simulink model "bike_model_v1_20190531_oldmodel_positionfeedback"  (R2016b)
settings: Solver=ode23s  StartTime=0.0  StopTime=sim_time  FixedStep=Ts_IMU  MaxStep=Ts  RelTol=1e-3
values from neighbouring files (symbols this model uses):
  A = [0      0            1 ... (first row only)    [bike_init_v1_20190528_oldmodel_positionfeedback_and_indicator.m]    (also in bike_init_v1_20190531_oldmodel_positionfeedback_and_indicator.m)
  A_kalman = [1 0 Ts 0; 0 1 0 Ts; 0 0 1 0; 0 0 0 1]    [bike_init_v1_20190528_oldmodel_positionfeedback_and_indicator.m]    (also in bike_init_v1_20190531_oldmodel_positionfeedback_and_indicator.m)
  a_real = b_real-0.77    (= 0.325)    [bike_init_v1_20190528_oldmodel_positionfeedback_and_indicator.m]    (also in bike_init_v1_20190531_oldmodel_positionfeedback_and_indicator.m)
  B = [0; 1; (a_real*v*sin(lambda_real))/(h_real*b_real)]    [bike_init_v1_20190528_oldmodel_positionfeedback_and_indicator.m]    (also in bike_init_v1_20190531_oldmodel_positionfeedback_and_indicator.m)
  B_kalman = [0 0 0 0; 0 0 0 0; 0 0 0 0; 0 0 0 0]    [bike_init_v1_20190528_oldmodel_positionfeedback_and_indicator.m]    (also in bike_init_v1_20190531_oldmodel_positionfeedback_and_indicator.m)
  b_model = 1.095    [bike_init_v1_20190528_oldmodel_positionfeedback_and_indicator.m]    (also in bike_init_v1_20190531_oldmodel_positionfeedback_and_indicator.m)
  b_real = 1.095    [bike_init_v1_20190528_oldmodel_positionfeedback_and_indicator.m]    (also in bike_init_v1_20190531_oldmodel_positionfeedback_and_indicator.m)
  C = eye(3)    [bike_init_v1_20190528_oldmodel_positionfeedback_and_indicator.m]    (also in bike_init_v1_20190531_oldmodel_positionfeedback_and_indicator.m)
  C_kalman = [1 0 0 0; 0 1 0 0; 0 0 1 0; 0 0 0 1]    [bike_init_v1_20190528_oldmodel_positionfeedback_and_indicator.m]    (also in bike_init_v1_20190531_oldmodel_positionfeedback_and_indicator.m)
  complementary = 0.985    [bike_init_v1_20190528_oldmodel_positionfeedback_and_indicator.m]    (also in bike_init_v1_20190531_oldmodel_positionfeedback_and_indicator.m)
  cumulative_dist_along_path = [0;cumsum(dist_from_vertex_to_vertex,1)]    [bike_init_v1_20190528_oldmodel_positionfeedback_and_indicator.m]    (also in bike_init_v1_20190531_oldmodel_positionfeedback_and_indicator.m)
  D = zeros(3,1)    [bike_init_v1_20190528_oldmodel_positionfeedback_and_indicator.m]    (also in bike_init_v1_20190531_oldmodel_positionfeedback_and_indicator.m)
  D_kalman = [0 0 0 0; 0 0 0 0; 0 0 0 0; 0 0 0 0]    [bike_init_v1_20190528_oldmodel_positionfeedback_and_indicator.m]    (also in bike_init_v1_20190531_oldmodel_positionfeedback_and_indicator.m)
  damp = 0.4    [bike_init_v1_20190528_oldmodel_positionfeedback_and_indicator.m]    (also in bike_init_v1_20190531_oldmodel_positionfeedback_and_indicator.m)
  Dead_Band = [0.055,-0.055,0.005]    [bike_init_v1_20190528_oldmodel_positionfeedback_and_indicator.m]    (also in bike_init_v1_20190531_oldmodel_positionfeedback_and_indicator.m)
  delay = 0.045    [bike_init_v1_20190528_oldmodel_positionfeedback_and_indicator.m]    (also in bike_init_v1_20190531_oldmodel_positionfeedback_and_indicator.m)
  delta_control = 1    [bike_init_v1_20190528_oldmodel_positionfeedback_and_indicator.m]    (also in bike_init_v1_20190531_oldmodel_positionfeedback_and_indicator.m)
  direct_control = 1    [bike_init_v1_20190528_oldmodel_positionfeedback_and_indicator.m]    (also in bike_init_v1_20190531_oldmodel_positionfeedback_and_indicator.m)
  filter_model = 1    [bike_init_v1_20190528_oldmodel_positionfeedback_and_indicator.m]    (also in bike_init_v1_20190531_oldmodel_positionfeedback_and_indicator.m)
  forward_motor_dynamics = 0    [bike_init_v1_20190528_oldmodel_positionfeedback_and_indicator.m]    (also in bike_init_v1_20190531_oldmodel_positionfeedback_and_indicator.m)
  fr_oscil = 1    [bike_init_v1_20190528_oldmodel_positionfeedback_and_indicator.m]    (also in bike_init_v1_20190531_oldmodel_positionfeedback_and_indicator.m)
  g = 9.81    [bike_init_v1_20190528_oldmodel_positionfeedback_and_indicator.m]    (also in bike_init_v1_20190531_oldmodel_positionfeedback_and_indicator.m)
  gain = 0.3    [bike_init_v1_20190528_oldmodel_positionfeedback_and_indicator.m]    (also in bike_init_v1_20190531_oldmodel_positionfeedback_and_indicator.m)
  h_real = 0.586    [bike_init_v1_20190528_oldmodel_positionfeedback_and_indicator.m]    (also in bike_init_v1_20190531_oldmodel_positionfeedback_and_indicator.m)
  IMU_height_model = 0.45    [bike_init_v1_20190528_oldmodel_positionfeedback_and_indicator.m]    (also in bike_init_v1_20190531_oldmodel_positionfeedback_and_indicator.m)
  IMU_height_real = 0.45    [bike_init_v1_20190528_oldmodel_positionfeedback_and_indicator.m]    (also in bike_init_v1_20190531_oldmodel_positionfeedback_and_indicator.m)
  initial_states = [deg2rad(0) deg2rad(0) deg2rad(0)]    [bike_init_v1_20190528_oldmodel_positionfeedback_and_indicator.m]    (also in bike_init_v1_20190531_oldmodel_positionfeedback_and_indicator.m = [deg2rad(2) deg2rad(0) deg2rad(0)])
  initial_x = path_x(1)+x_ini_diff    [bike_init_v1_20190528_oldmodel_positionfeedback_and_indicator.m]    (also in bike_init_v1_20190531_oldmodel_positionfeedback_and_indicator.m = 0)
  initial_y = radius+y_ini_diff    (= 20)    [bike_init_v1_20190528_oldmodel_positionfeedback_and_indicator.m]    (also in bike_init_v1_20190531_oldmodel_positionfeedback_and_indicator.m = 0)
  input_velocity = 7    [bike_init_v1_20190528_oldmodel_positionfeedback_and_indicator.m]    (also in bike_init_v1_20190531_oldmodel_positionfeedback_and_indicator.m = 3)
  K_full_dis = zeros(length(velocity_lqr),3)    [bike_init_v1_20190528_oldmodel_positionfeedback_and_indicator.m]    (also in bike_init_v1_20190531_oldmodel_positionfeedback_and_indicator.m)
  lambda_model = deg2rad(70)    [bike_init_v1_20190528_oldmodel_positionfeedback_and_indicator.m]    (also in bike_init_v1_20190531_oldmodel_positionfeedback_and_indicator.m)
  lambda_real = deg2rad(70)    [bike_init_v1_20190528_oldmodel_positionfeedback_and_indicator.m]    (also in bike_init_v1_20190531_oldmodel_positionfeedback_and_indicator.m)
  lat_control = 1    [bike_init_v1_20190528_oldmodel_positionfeedback_and_indicator.m]    (also in bike_init_v1_20190531_oldmodel_positionfeedback_and_indicator.m)
  look_ahead = 0    [bike_init_v1_20190528_oldmodel_positionfeedback_and_indicator.m]    (also in bike_init_v1_20190531_oldmodel_positionfeedback_and_indicator.m)
  max_handlebar = 40*(pi/180)    (= 0.698131700798)    [bike_init_v1_20190528_oldmodel_positionfeedback_and_indicator.m]    (also in bike_init_v1_20190531_oldmodel_positionfeedback_and_indicator.m)
  max_roll = pi/2    (= 1.57079632679)    [bike_init_v1_20190528_oldmodel_positionfeedback_and_indicator.m]    (also in bike_init_v1_20190531_oldmodel_positionfeedback_and_indicator.m)
  max_steering_motor_acc = inf    [bike_init_v1_20190528_oldmodel_positionfeedback_and_indicator.m]    (also in bike_init_v1_20190531_oldmodel_positionfeedback_and_indicator.m)
  max_steering_motor_speed = 7.5    [bike_init_v1_20190528_oldmodel_positionfeedback_and_indicator.m]    (also in bike_init_v1_20190531_oldmodel_positionfeedback_and_indicator.m)
  min_handlebar = -max_handlebar    (= -0.698131700798)    [bike_init_v1_20190528_oldmodel_positionfeedback_and_indicator.m]    (also in bike_init_v1_20190531_oldmodel_positionfeedback_and_indicator.m)
  min_roll = - max_roll    (= -1.57079632679)    [bike_init_v1_20190528_oldmodel_positionfeedback_and_indicator.m]    (also in bike_init_v1_20190531_oldmodel_positionfeedback_and_indicator.m)
  min_steering_motor_acc = -inf    [bike_init_v1_20190528_oldmodel_positionfeedback_and_indicator.m]    (also in bike_init_v1_20190531_oldmodel_positionfeedback_and_indicator.m)
  min_steering_motor_speed = -7.5    [bike_init_v1_20190528_oldmodel_positionfeedback_and_indicator.m]    (also in bike_init_v1_20190531_oldmodel_positionfeedback_and_indicator.m)
  noise = 1    [bike_init_v1_20190528_oldmodel_positionfeedback_and_indicator.m]    (also in bike_init_v1_20190531_oldmodel_positionfeedback_and_indicator.m)
  noise_encoder = 1e-7    (= 1e-07)    [bike_init_v1_20190528_oldmodel_positionfeedback_and_indicator.m]    (also in bike_init_v1_20190531_oldmodel_positionfeedback_and_indicator.m)
  noise_hall = 0.01    [bike_init_v1_20190528_oldmodel_positionfeedback_and_indicator.m]    (also in bike_init_v1_20190531_oldmodel_positionfeedback_and_indicator.m = 0.0031)
  noise_pos_meas = 0.51    [bike_init_v1_20190528_oldmodel_positionfeedback_and_indicator.m]    (also in bike_init_v1_20190531_oldmodel_positionfeedback_and_indicator.m)
  oscillations_roll = 0    [bike_init_v1_20190528_oldmodel_positionfeedback_and_indicator.m]    (also in bike_init_v1_20190531_oldmodel_positionfeedback_and_indicator.m)
  oscillations_steer = 0    [bike_init_v1_20190528_oldmodel_positionfeedback_and_indicator.m]    (also in bike_init_v1_20190531_oldmodel_positionfeedback_and_indicator.m)
  parameters_model = [g h_model b_model a_model lambda_model c_model]    [bike_init_v1_20190528_oldmodel_positionfeedback_and_indicator.m]    (also in bike_init_v1_20190531_oldmodel_positionfeedback_and_indicator.m)
  parameters_real = [g h_real b_real a_real lambda_real c_real]    [bike_init_v1_20190528_oldmodel_positionfeedback_and_indicator.m]    (also in bike_init_v1_20190531_oldmodel_positionfeedback_and_indicator.m)
  path_tracking = 0    [bike_init_v1_20190528_oldmodel_positionfeedback_and_indicator.m]    (also in bike_init_v1_20190531_oldmodel_positionfeedback_and_indicator.m)
  path_x = [path_x1 path_x2 path_x3]    [bike_init_v1_20190528_oldmodel_positionfeedback_and_indicator.m]    (also in bike_init_v1_20190531_oldmodel_positionfeedback_and_indicator.m)
  path_y = [path_y1 path_y2 path_y3]    [bike_init_v1_20190528_oldmodel_positionfeedback_and_indicator.m]    (also in bike_init_v1_20190531_oldmodel_positionfeedback_and_indicator.m)
  plant_model = 1    [bike_init_v1_20190528_oldmodel_positionfeedback_and_indicator.m]    (also in bike_init_v1_20190531_oldmodel_positionfeedback_and_indicator.m)
  R_kalman = [noise_pos_meas 0 0 0; 0 noise_pos_meas 0 0; 0 0 noise_hall 0; 0 0 0 noise_hall]    [bike_init_v1_20190528_oldmodel_positionfeedback_and_indicator.m]    (also in bike_init_v1_20190531_oldmodel_positionfeedback_and_indicator.m)
  roll_rate_coef = 0.9    [bike_init_v1_20190528_oldmodel_positionfeedback_and_indicator.m]    (also in bike_init_v1_20190531_oldmodel_positionfeedback_and_indicator.m)
  steering_motor_limitations = 1    [bike_init_v1_20190528_oldmodel_positionfeedback_and_indicator.m]    (also in bike_init_v1_20190531_oldmodel_positionfeedback_and_indicator.m)
  sys_con = ss(A,B,C,D)    [bike_init_v1_20190528_oldmodel_positionfeedback_and_indicator.m]    (also in bike_init_v1_20190531_oldmodel_positionfeedback_and_indicator.m)
  sys_dis = c2d(sys_con,Ts)    [bike_init_v1_20190528_oldmodel_positionfeedback_and_indicator.m]    (also in bike_init_v1_20190531_oldmodel_positionfeedback_and_indicator.m)
  Ts = 0.04    [bike_init_v1_20190528_oldmodel_positionfeedback_and_indicator.m]    (also in bike_init_v1_20190531_oldmodel_positionfeedback_and_indicator.m)
  Ts_IMU = 0.04    [bike_init_v1_20190528_oldmodel_positionfeedback_and_indicator.m]    (also in bike_init_v1_20190531_oldmodel_positionfeedback_and_indicator.m)
  velocity_lqr = [velocity_lqr-0.1 velocity_lqr velocity_lqr+0.1]    [bike_init_v1_20190528_oldmodel_positionfeedback_and_indicator.m]    (also in bike_init_v1_20190531_oldmodel_positionfeedback_and_indicator.m)
  velocity_wave_amp = 0.5    [bike_init_v1_20190528_oldmodel_positionfeedback_and_indicator.m]    (also in bike_init_v1_20190531_oldmodel_positionfeedback_and_indicator.m)
  velocity_wave_freq = 0.3*2*pi    (= 1.88495559215)    [bike_init_v1_20190528_oldmodel_positionfeedback_and_indicator.m]    (also in bike_init_v1_20190531_oldmodel_positionfeedback_and_indicator.m)
undefined symbols (not defined in the file or in its folder): Continuous, curvature, Time
libraries: simulink x13, mpclib x2, dspsigops x2, simulink_extras x1, ctrlSharedLib x1
(part 1 of 2)
settings Model: Creator=Boaz Ash  LastModifiedBy=maximefeingesicht
settings DebuggingCC: UnconnectedInputMsg=none  UnconnectedOutputMsg=none  UnconnectedLineMsg=none

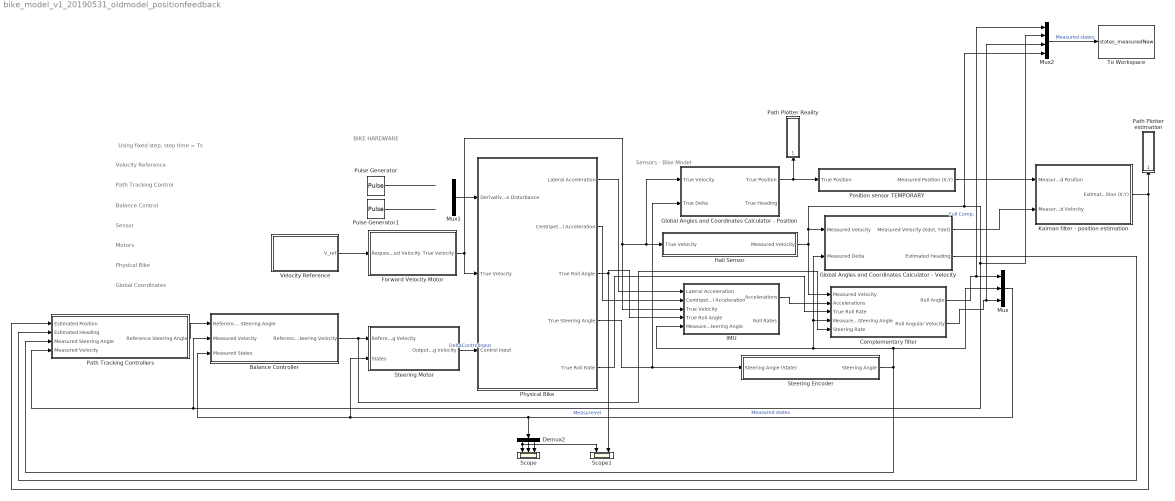
== system bike_model_v1_20190531_oldmodel_positionfeedback ==
  note: Using fixed step, step time = Ts
  note: BIKE HARDWARE
  note: Velocity Reference
  note: Sensor
  note: Sensors - Bike Model
  note: Balance Control
  note: Motors
  note: Physical Bike
  note: Path Tracking Control
  note: Global Coordinates
  Balance Controller : Subsystem  TreatAsAtomicUnit=on  SystemSampleTime=Ts
  Complementary filter : Subsystem  SystemSampleTime=Ts_IMU
  Demux2 : Demux  Outputs=3
  Forward Velocity Motor : Subsystem
  Global Angles and Coordinates Calculator - Position : Subsystem  SystemSampleTime=Ts
  Global Angles and Coordinates Calculator - Velocity : Subsystem  SystemSampleTime=Ts
  Hall Sensor : Subsystem  TreatAsAtomicUnit=on  SystemSampleTime=Ts
  IMU : Subsystem  TreatAsAtomicUnit=on
  "Kalman filter - position estimation " : Subsystem  SystemSampleTime=Ts
  Mux : Mux  Inputs=3
  Mux1 : Mux  Inputs=3
  Mux2 : Mux
  Path Plotter Reality : Subsystem  SystemSampleTime=Ts
  Path Plotter estimation : Subsystem  SystemSampleTime=Ts
  Path Tracking Controllers : Subsystem
  Physical Bike : Subsystem
  Position sensor TEMPORARY : Subsystem  TreatAsAtomicUnit=on  SystemSampleTime=Ts
  Pulse Generator : DiscretePulseGenerator  PulseType=Time based  Amplitude=pi/36  Period=100  PhaseDelay=1
  Pulse Generator1 : DiscretePulseGenerator  PulseType=Time based  Amplitude=-deg2rad(30)  Period=10  PulseWidth=10  PhaseDelay=1
  Scope : Scope  NumInputPorts=3
  Scope1 : Scope  NumInputPorts=2
  Steering Encoder : Subsystem  TreatAsAtomicUnit=on  SystemSampleTime=Ts
  Steering Motor : Subsystem
  To Workspace : ToWorkspace  VariableName=states_measuredNew  SaveFormat=Timeseries  SampleTime=-1
  Velocity Reference : Subsystem
  wires:
  Mux1/1 -> Physical Bike/1(Derivative Disturbance)
  Velocity Reference/1(V_ref) -> Forward Velocity Motor/1(Requested Velocity)
  Demux2/2 -> Scope/2
  Demux2/3 -> Scope/3
  Forward Velocity Motor/1(True Velocity) -> IMU/3(True Velocity), Global Angles and Coordinates Calculator - Position/1(True Velocity), Hall Sensor/1(True Velocity), Physical Bike/2(True Velocity)
  Pulse Generator/1 -> ?
  Physical Bike/4(True Steering Angle) -> Global Angles and Coordinates Calculator - Position/2(True Delta), Steering Encoder/1(Steering Angle (State))
  Pulse Generator1/1 -> ?
  "Kalman filter - position estimation "/1(Estimated Position (X,Y)) -> Path Tracking Controllers/1(Estimated Position), Path Plotter estimation/1(Position)
  Global Angles and Coordinates Calculator - Velocity/2(Estimated Heading) -> Path Tracking Controllers/2(Estimated Heading)
  Path Tracking Controllers/1(Reference Steering Angle) -> Balance Controller/1(Reference Steering Angle)
  Balance Controller/1(Reference Steering Velocity) -> Complementary filter/5(Steering Rate), Steering Motor/1(Reference Steering Velocity)
  Demux2/1 -> Scope1/1, Scope/1
  Physical Bike/1(Lateral Acceleration) -> IMU/1(Lateral Acceleration)
  Physical Bike/2(Centripetal Acceleration) -> IMU/2(Centripetal Acceleration)
  Mux/1 -> Demux2/1, Steering Motor/2(States), Balance Controller/3(Measured States)  "Measured states"
  Physical Bike/5(True Roll Rate) -> Complementary filter/3(True Roll Rate)
  Physical Bike/3(True Roll Angle) -> IMU/4(True Roll Angle), Scope1/2
  Steering Motor/1(Output Steering Velocity) -> Physical Bike/3(Control Input)  "DeltaControlInput"
  Steering Encoder/1(Steering Angle) -> Global Angles and Coordinates Calculator - Velocity/2(Measured Delta), Complementary filter/4(Measured Steering Angle), IMU/5(Measured Steering Angle), Mux/2, Path Tracking Controllers/3(Measured Steering Angle)
  IMU/1(Accelerations) -> Complementary filter/2(Accelerations)
  Position sensor TEMPORARY/1("Measured Position (X,Y) ") -> "Kalman filter - position estimation "/1("Measured Position ")
  Global Angles and Coordinates Calculator - Position/1(True Position) -> Path Plotter Reality/1(Position), Position sensor TEMPORARY/1(True Position)
  Global Angles and Coordinates Calculator - Velocity/1("Measured Velocity (Xdot, Ydot)") -> "Kalman filter - position estimation "/2(Measured Velocity)
  Complementary filter/2(Roll Angular Velocity) -> Mux2/3, Mux/3
  Complementary filter/1(Roll Angle) -> Mux2/1, Mux/1  "Full Comp."
  Hall Sensor/1(Measured Velocity) -> Mux2/4, Path Tracking Controllers/4(Measured Velocity), Balance Controller/2(Measured Velocity), Mux2/2, Global Angles and Coordinates Calculator - Velocity/1(Measured Velocity), Complementary filter/1(Measured Velocity)  "MeasureVel"
  Mux2/1 -> To Workspace/1  "Measured states"

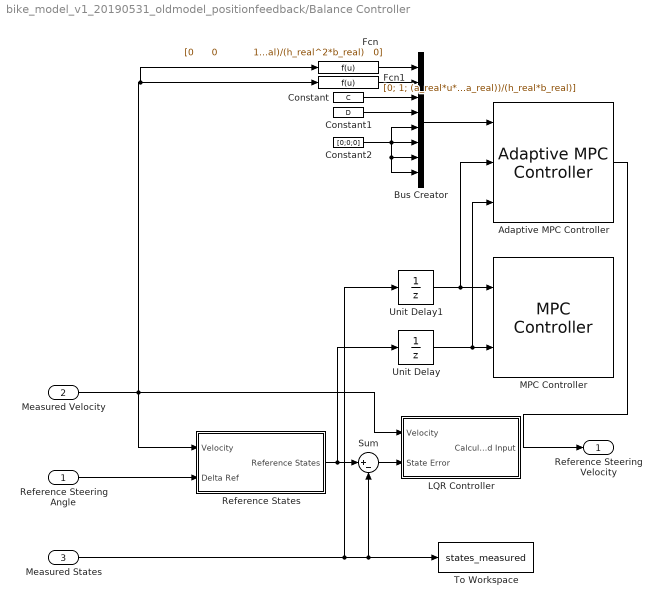
== system bike_model_v1_20190531_oldmodel_positionfeedback/Balance Controller ==
  Reference Steering Angle : Inport
  Measured Velocity : Inport  Port=2
  Measured States : Inport  Port=3
  Adaptive MPC Controller : mpclib/Adaptive MPC Controller  SCDEnableBlockLinearizationSpecification=on  mpcobj=mpcObj  md_inport=off  mv_inport=off  cost_outport=off  return_sequence=off  return_qpstatus=off  return_state=off  state_inport=off  isltv_plant=off  lims_inport=off  ywt_inport=off  uwt_inport=off  duwt_inport=off  rhoeps_inport=off  uref_inport=off  BlockDataType=double  SampleTimeInherited=off  switch_inport=off
  Bus Creator : BusCreator  Inputs='A','B','C','D','X','Y','U','DX'
  Constant : Constant  Value=C  SampleTime=Ts
  Constant1 : Constant  Value=D  SampleTime=Ts
  Constant2 : Constant  Value=[0;0;0]  SampleTime=Ts
  Fcn : Fcn  Expr=|
      | [0      0            1;
      |              0      0            0;
      |              g/h_real    sin(lambda_real)*(h_real*u^2-g*a_real*c_real)/(h_real^2*b_real)   0]
  Fcn1 : Fcn  Expr=[0; 1; (a_real*u*sin(lambda_real))/(h_real*b_real)]
  LQR Controller : Subsystem  TreatAsAtomicUnit=on  SystemSampleTime=Ts
  MPC Controller : mpclib/MPC Controller  SCDEnableBlockLinearizationSpecification=on  mpcobj=mpcObj  is_multiple=0  enable_value=0  return_u0=off  ref_from_ws=off  ref_signal_name=[]  ref_preview=off  md_from_ws=off  md_signal_name=[]  md_preview=off  from_project=off  project_file=MPCtask.mat  md_inport=off  mv_inport=off  cost_outport=off  return_sequence=off  return_qpstatus=off  return_state=off  state_inport=off  lims_inport=off  ywt_inport=off  is_designfromscratch=0  uwt_inport=off  duwt_inport=off  rhoeps_inport=off  uref_inport=off  n_ts=0.04  n_mv=1  n_md=0  n_ud=0  n_mo=3  n_uo=0  BlockDataType=double  SampleTimeInherited=off  switch_inport=off
  Reference States : Subsystem  SystemSampleTime=Ts
  Sum : Sum  Inputs=|+-
  To Workspace : ToWorkspace  VariableName=states_measured  SaveFormat=Timeseries  SampleTime=-1
  Unit Delay : UnitDelay  InitialCondition=[0 0 0]  SampleTime=-1
  Unit Delay1 : UnitDelay  InitialCondition=[0 0 0]  SampleTime=-1
  Reference Steering Velocity : Outport
  wires:
  Reference States/1(Reference States) -> Unit Delay/1, Sum/1
  Sum/1 -> LQR Controller/2(State Error)
  Adaptive MPC Controller/1 -> Reference Steering Velocity/1
  Reference Steering Angle/1 -> Reference States/2(Delta Ref)
  Measured Velocity/1 -> Fcn/1, Fcn1/1, Reference States/1(Velocity), LQR Controller/1(Velocity)
  Unit Delay/1 -> Adaptive MPC Controller/3, MPC Controller/2
  Measured States/1 -> Unit Delay1/1, To Workspace/1, Sum/2
  Unit Delay1/1 -> Adaptive MPC Controller/2, MPC Controller/1
  Bus Creator/1 -> Adaptive MPC Controller/1
  Fcn1/1 -> Bus Creator/2
  Fcn/1 -> Bus Creator/1
  Constant/1 -> Bus Creator/3
  Constant1/1 -> Bus Creator/4
  Constant2/1 -> Bus Creator/7, Bus Creator/8, Bus Creator/6, Bus Creator/5

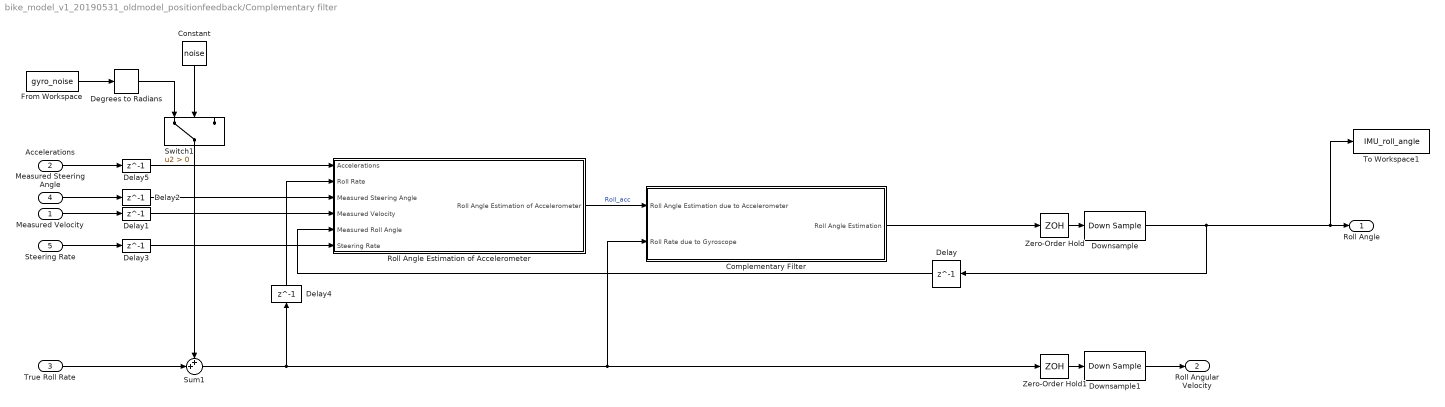
== system bike_model_v1_20190531_oldmodel_positionfeedback/Complementary filter ==
  Measured Velocity : Inport
  Accelerations : Inport  Port=2
  True Roll Rate : Inport  Port=3
  Measured Steering Angle : Inport  Port=4
  Steering Rate : Inport  Port=5
  Complementary Filter : Subsystem  TreatAsAtomicUnit=on  SystemSampleTime=Ts_IMU
  Constant : Constant  Value=noise
  Degrees to Radians : simulink_extras/Transformations/Degrees to Radians
  Delay{,1..2,4..5} (5 alike) : Delay  DelayLength=1
  Delay3 : Delay  DelayLength=1  SampleTime=Ts_IMU
  Downsample : DownSample  N=Ts/Ts_IMU  RateOptions=Allow multirate processing
  Downsample1 : DownSample  N=Ts/Ts_IMU  RateOptions=Allow multirate processing
  From Workspace : FromWorkspace  VariableName=gyro_noise  SampleTime=0
  Roll Angle Estimation of Accelerometer : Subsystem
  Sum1 : Sum  Inputs=++|
  Switch1 : Switch  Criteria=u2 > Threshold
  To Workspace1 : ToWorkspace  VariableName=IMU_roll_angle  SaveFormat=Structure  SampleTime=-1
  Zero-Order Hold : ZeroOrderHold  SampleTime=Ts_IMU
  Zero-Order Hold1 : ZeroOrderHold  SampleTime=Ts_IMU
  Roll Angle : Outport
  Roll Angular Velocity : Outport  Port=2
  wires:
  Constant/1 -> Switch1/2
  True Roll Rate/1 -> Sum1/2
  Roll Angle Estimation of Accelerometer/1(Roll Angle Estimation of Accelerometer) -> Complementary Filter/1(Roll Angle Estimation due to Accelerometer)  "Roll_acc"
  Switch1/1 -> Sum1/1
  Sum1/1 -> Zero-Order Hold1/1, Complementary Filter/2(Roll Rate due to Gyroscope), Delay4/1
  Zero-Order Hold/1 -> Downsample/1
  Zero-Order Hold1/1 -> Downsample1/1
  Accelerations/1 -> Delay5/1
  Measured Steering Angle/1 -> Delay2/1
  Measured Velocity/1 -> Delay1/1
  Delay/1 -> Roll Angle Estimation of Accelerometer/5(Measured Roll Angle)
  Delay1/1 -> Roll Angle Estimation of Accelerometer/4(Measured Velocity)
  Delay2/1 -> Roll Angle Estimation of Accelerometer/3(Measured Steering Angle)
  Steering Rate/1 -> Delay3/1
  Delay3/1 -> Roll Angle Estimation of Accelerometer/6(Steering Rate)
  Delay4/1 -> Roll Angle Estimation of Accelerometer/2(Roll Rate)
  Delay5/1 -> Roll Angle Estimation of Accelerometer/1(Accelerations)
  Complementary Filter/1(Roll Angle Estimation) -> Zero-Order Hold/1
  From Workspace/1 -> Degrees to Radians/1
  Degrees to Radians/1 -> Switch1/1
  Downsample1/1 -> Roll Angular Velocity/1
  Downsample/1 -> To Workspace1/1, Roll Angle/1, Delay/1

== system bike_model_v1_20190531_oldmodel_positionfeedback/Forward Velocity Motor ==
  note: Add limit for acceleration/deceleration
      | Add min speed of 1.69 m/s (3600 rpm motor speed) limitation
      | Add min speed of 8.20 m/s (18000 rpm motor speed) limitation
      | Add deadband and delay
  Requested Velocity : Inport
  Constant : Constant  Value=forward_motor_dynamics
  Rate Limiter : RateLimiter  RisingSlewLimit=inf  FallingSlewLimit=-inf  SampleTimeMode=inherited
  Saturation : Saturate  UpperLimit=inf  LowerLimit=0
  Scope : Scope
  Sine Wave : Sin  Amplitude=velocity_wave_amp  Frequency=velocity_wave_freq  SampleTime=0
  Sum : Sum  Inputs=|++
  Switch : Switch  Criteria=u2 > Threshold
  Transfer Fcn : TransferFcn  Numerator=[-0.2156 0.556]  Denominator=[1 1.675 0.5558]
  True Velocity : Outport
  wires:
  Requested Velocity/1 -> Transfer Fcn/1, Switch/3
  Transfer Fcn/1 -> Rate Limiter/1
  Switch/1 -> Sum/1
  Constant/1 -> Switch/2
  Saturation/1 -> Switch/1
  Rate Limiter/1 -> Saturation/1
  Sum/1 -> Scope/1, True Velocity/1
  Sine Wave/1 -> Sum/2

== system bike_model_v1_20190531_oldmodel_positionfeedback/Global Angles and Coordinates Calculator - Position ==
  True Velocity : Inport
  True Delta : Inport  Port=2
  Gain1 : Gain  Gain=sin(lambda_model)
  Measured Bike Angles to Global Angles : Subsystem
  Measured Global Angles to Global Coordinates : Subsystem
  Sum : Sum  Inputs=++|
  To Workspace : ToWorkspace  VariableName=pos_true  SaveFormat=Timeseries  SampleTime=-1
  True Position : Outport
  True Heading : Outport  Port=2
  wires:
  True Delta/1 -> Gain1/1
  Measured Bike Angles to Global Angles/1(psi) -> Sum/2, Measured Global Angles to Global Coordinates/2(Psi)
  Gain1/1 -> Measured Bike Angles to Global Angles/2(Steering Angle)
  Sum/1 -> True Heading/1
  Measured Bike Angles to Global Angles/2(beta) -> Sum/1, Measured Global Angles to Global Coordinates/3(Beta)
  Measured Global Angles to Global Coordinates/1("Position (X, Y)") -> To Workspace/1, True Position/1
  True Velocity/1 -> Measured Bike Angles to Global Angles/1(Velocity), Measured Global Angles to Global Coordinates/1(Velocity)

== system bike_model_v1_20190531_oldmodel_positionfeedback/Global Angles and Coordinates Calculator - Velocity ==
  Measured Velocity : Inport
  Measured Delta : Inport  Port=2
  Gain1 : Gain  Gain=sin(lambda_model)
  Integrator2 : Integrator
  Measured Bike Angles to Global Angles : Subsystem
  Measured Global Angles to Global Coordinates : Subsystem
  Sum : Sum  Inputs=++|
  To Workspace1 : ToWorkspace  VariableName=pos_vel_int  SaveFormat=Timeseries  SampleTime=-1
  "Measured Velocity (Xdot, Ydot)" : Outport
  Estimated Heading : Outport  Port=2
  wires:
  Measured Delta/1 -> Gain1/1
  Measured Bike Angles to Global Angles/1(psi) -> Sum/2, Measured Global Angles to Global Coordinates/2(Psi)
  Gain1/1 -> Measured Bike Angles to Global Angles/2(Steering Angle)
  Sum/1 -> Estimated Heading/1
  Measured Bike Angles to Global Angles/2(beta) -> Measured Global Angles to Global Coordinates/3(Beta), Sum/1
  Measured Velocity/1 -> Measured Bike Angles to Global Angles/1(Velocity), Measured Global Angles to Global Coordinates/1(Velocity)
  Measured Global Angles to Global Coordinates/1("Velocity (Xdot, Ydot)") -> Integrator2/1, "Measured Velocity (Xdot, Ydot)"/1
  Integrator2/1 -> To Workspace1/1

== system bike_model_v1_20190531_oldmodel_positionfeedback/Hall Sensor ==
  True Velocity : Inport
  Constant : Constant  Value=noise
  Noise on hall sensor : RandomNumber  Variance=noise_hall  SampleTime=Ts
  Saturate Signal : Switch  Criteria=u2 > Threshold
  Sum : Sum  Inputs=++|
  Switch : Switch  Criteria=u2 > Threshold
  To Workspace3 : ToWorkspace  VariableName=vel_meas  SaveFormat=Timeseries  SampleTime=-1
  Velocity Lower Bound : simulink/Model Verification/Check Static  Lower Bound  Description=0.6 <= u  min=0.6  min_included=on  enabled=on  stopWhenAssertionFail=off  export=on  icon=graphic
  Zero : Constant  Value=0
  Zero-Order Hold : ZeroOrderHold  SampleTime=Ts
  Measured Velocity : Outport
  wires:
  Constant/1 -> Switch/2
  Switch/1 -> Saturate Signal/1, Velocity Lower Bound/1
  Noise on hall sensor/1 -> Sum/1
  Sum/1 -> Switch/1
  Zero/1 -> Saturate Signal/3
  Velocity Lower Bound/1 -> Saturate Signal/2
  Saturate Signal/1 -> Zero-Order Hold/1
  Zero-Order Hold/1 -> Measured Velocity/1, To Workspace3/1
  True Velocity/1 -> Switch/3, Sum/2

== system bike_model_v1_20190531_oldmodel_positionfeedback/IMU ==
  Lateral Acceleration : Inport
  Centripetal Acceleration : Inport  Port=2
  True Velocity : Inport  Port=3
  True Roll Angle : Inport  Port=4
  Measured Steering Angle : Inport  Port=5
  IMU : Subsystem
  Accelerations : Outport
  Roll Rates : Outport  Port=2
  wires:
  True Velocity/1 -> IMU/3(True Velocity)
  True Roll Angle/1 -> IMU/4(True Roll Angle)
  Measured Steering Angle/1 -> IMU/5(Measured Steering Angle)
  Lateral Acceleration/1 -> IMU/1(Lateral Acceleration)
  Centripetal Acceleration/1 -> IMU/2(Centripetal Acceleration)
  IMU/1(Accelerations) -> Accelerations/1
  IMU/2(Roll Rates) -> Roll Rates/1

== system bike_model_v1_20190531_oldmodel_positionfeedback/Kalman filter - position estimation  ==
  note: y_k
  note: Measurements
  "Measured Position " : Inport
  Measured Velocity : Inport  Port=2
  Demux : Demux  Outputs=2
  "Kalman Filter " : ctrlSharedLib/Kalman Filter  TimeDomain=Continuous-Time  UseCurrentEstimator=on  ModelSource=Individual A, B, C, D matrices  ModelSourceVariable=ss(0.95,1,1,0,1)  A=A_kalman  B=B_kalman  C=C_kalman  D=D_kalman  NumberOfStates=1  NumberOfInputs=1  NumberOfOutputs=1  InitialEstimateSource=Dialog  X0=0  P0=10  UseK=off  UseGH=off  NumberOfProcessNoiseInputs=1  G=1  TimeInvariantG=on  H=0  TimeInvariantH=on  Q=Q_kalman  TimeInvariantQ=on  R=R_kalman  TimeInvariantR=on  N=0  TimeInvariantN=on  AddInputPort=on  AddEnablePort=off  ExternalReset=none  OutputEstimatedY=off  OutputP=off  Ts=Ts
  Mux : Mux  Inputs=2
  Estimated Position (X,Y) : Outport
  wires:
  Measured Velocity/1 -> Mux/2
  Mux/1 -> "Kalman Filter "/2
  "Measured Position "/1 -> Mux/1
  "Kalman Filter "/1 -> Demux/1
  Demux/1 -> Estimated Position (X,Y)/1

== system bike_model_v1_20190531_oldmodel_positionfeedback/Path Plotter Reality ==
  Position : Inport
  Demux : Demux  Outputs=2
  To Workspace : ToWorkspace  VariableName=X_BIKE  SaveFormat=Timeseries  SampleTime=Ts
  To Workspace1 : ToWorkspace  VariableName=Y_BIKE  SaveFormat=Timeseries  SampleTime=Ts
  XY Graph : simulink/Sinks/XY Graph  Commented=on  xmin=min(path_x)-5  xmax=max(path_x)+5  ymin=min(path_y)-5  ymax=max(path_y)+5  st=-1
  wires:
  Demux/1 -> XY Graph/1, To Workspace/1  "X"
  Demux/2 -> XY Graph/2, To Workspace1/1  "Y"
  Position/1 -> Demux/1

== system bike_model_v1_20190531_oldmodel_positionfeedback/Path Plotter estimation ==
  Position : Inport
  Demux : Demux  Outputs=2
  To Workspace : ToWorkspace  VariableName=X_BIKE_estim  SaveFormat=Timeseries  SampleTime=Ts
  To Workspace1 : ToWorkspace  VariableName=Y_BIKE_estim  SaveFormat=Timeseries  SampleTime=Ts
  XY Graph : simulink/Sinks/XY Graph  Commented=on  xmin=min(path_x)-5  xmax=max(path_x)+5  ymin=min(path_y)-5  ymax=max(path_y)+5  st=-1
  wires:
  Demux/1 -> XY Graph/1, To Workspace/1  "X"
  Demux/2 -> XY Graph/2, To Workspace1/1  "Y"
  Position/1 -> Demux/1

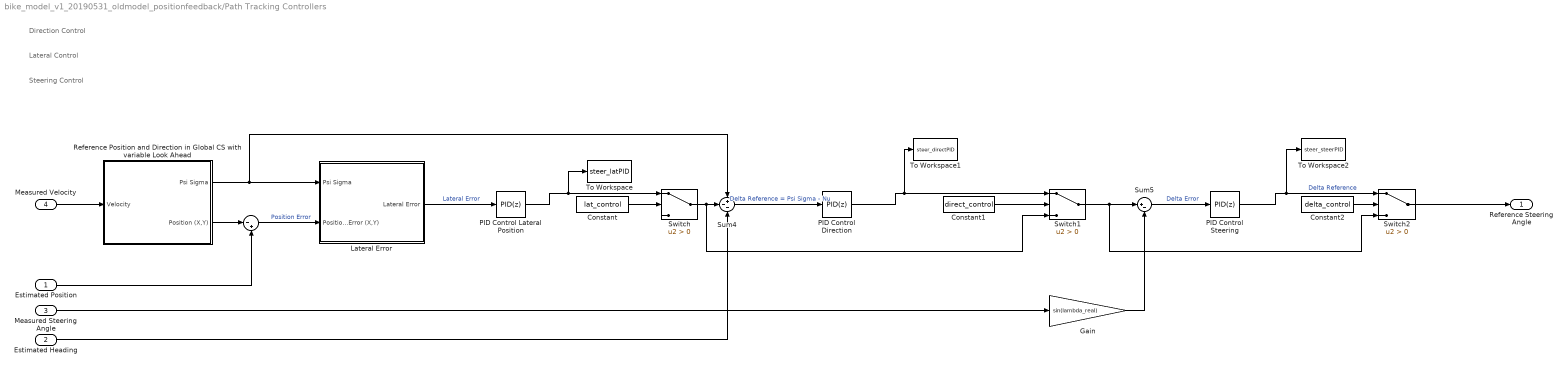
== system bike_model_v1_20190531_oldmodel_positionfeedback/Path Tracking Controllers ==
  note: Direction Control
  note: Lateral Control
  note: Steering Control
  Estimated Position : Inport
  Estimated Heading : Inport  Port=2
  Measured Steering Angle : Inport  Port=3
  Measured Velocity : Inport  Port=4
  " " : Sum  Inputs=|-+
  Constant : Constant  Value=lat_control
  Constant1 : Constant  Value=direct_control
  Constant2 : Constant  Value=delta_control
  Gain : Gain  Gain=sin(lambda_real)
  Lateral Error : Subsystem  SystemSampleTime=Ts
  PID Control Lateral Position : simulink/Continuous/PID Controller  Controller=PID  TimeDomain=Discrete-time  SampleTime=Ts  IntegratorMethod=Forward Euler  FilterMethod=Forward Euler  Form=Parallel  UseFilter=on  ControllerParametersSource=internal  P=0.05  I=0.01  D=0  N=100  InitialConditionSource=internal  InitialConditionForIntegrator=0  InitialConditionForFilter=0  ExternalReset=none  LimitOutput=off  UpperSaturationLimit=inf  LowerSaturationLimit=-inf  LinearizeAsGain=on  AntiWindupMode=none  Kb=1  TrackingMode=off  Kt=1  PParamMin=[]  PParamMax=[]  IParamMin=[]  IParamMax=[]  DParamMin=[]  DParamMax=[]  NParamMin=[]  NParamMax=[]  KbParamMin=[]  KbParamMax=[]  KtParamMin=[]  KtParamMax=[]  POutMin=[]  POutMax=[]  IOutMin=[]  IOutMax=[]  DOutMin=[]  DOutMax=[]  NOutMin=[]  NOutMax=[]  KbOutMin=[]  KbOutMax=[]  KtOutMin=[]  KtOutMax=[]  IntegratorOutMin=[]  IntegratorOutMax=[]  FilterOutMin=[]  FilterOutMax=[]  SumOutMin=[]  SumOutMax=[]  SumI1OutMin=[]  SumI1OutMax=[]  SumI2OutMin=[]  SumI2OutMax=[]  SumI3OutMin=[]  SumI3OutMax=[]  SumDOutMin=[]  SumDOutMax=[]  SaturationOutMin=[]  SaturationOutMax=[]  IntegratorContinuousStateAttributes=''  IntegratorStateMustResolveToSignalObject=off  IntegratorRTWStateStorageClass=Auto  FilterContinuousStateAttributes=''  FilterStateMustResolveToSignalObject=off  FilterRTWStateStorageClass=Auto  DifferentiatorICPrevScaledInput=0  DifferentiatorOutMin=[]  DifferentiatorOutMax=[]
  PID Control Direction : simulink/Continuous/PID Controller  Controller=PID  TimeDomain=Discrete-time  SampleTime=Ts  IntegratorMethod=Forward Euler  FilterMethod=Forward Euler  Form=Parallel  UseFilter=on  ControllerParametersSource=internal  P=0.6  I=0.5  D=0  N=100  InitialConditionSource=internal  InitialConditionForIntegrator=0  InitialConditionForFilter=0  ExternalReset=none  LimitOutput=off  UpperSaturationLimit=inf  LowerSaturationLimit=-inf  LinearizeAsGain=on  AntiWindupMode=none  Kb=1  TrackingMode=off  Kt=1  PParamMin=[]  PParamMax=[]  IParamMin=[]  IParamMax=[]  DParamMin=[]  DParamMax=[]  NParamMin=[]  NParamMax=[]  KbParamMin=[]  KbParamMax=[]  KtParamMin=[]  KtParamMax=[]  POutMin=[]  POutMax=[]  IOutMin=[]  IOutMax=[]  DOutMin=[]  DOutMax=[]  NOutMin=[]  NOutMax=[]  KbOutMin=[]  KbOutMax=[]  KtOutMin=[]  KtOutMax=[]  IntegratorOutMin=[]  IntegratorOutMax=[]  FilterOutMin=[]  FilterOutMax=[]  SumOutMin=[]  SumOutMax=[]  SumI1OutMin=[]  SumI1OutMax=[]  SumI2OutMin=[]  SumI2OutMax=[]  SumI3OutMin=[]  SumI3OutMax=[]  SumDOutMin=[]  SumDOutMax=[]  SaturationOutMin=[]  SaturationOutMax=[]  IntegratorContinuousStateAttributes=''  IntegratorStateMustResolveToSignalObject=off  IntegratorRTWStateStorageClass=Auto  FilterContinuousStateAttributes=''  FilterStateMustResolveToSignalObject=off  FilterRTWStateStorageClass=Auto  DifferentiatorICPrevScaledInput=0  DifferentiatorOutMin=[]  DifferentiatorOutMax=[]
  PID Control Steering : simulink/Continuous/PID Controller  Controller=PID  TimeDomain=Discrete-time  SampleTime=Ts  IntegratorMethod=Forward Euler  FilterMethod=Forward Euler  Form=Parallel  UseFilter=on  ControllerParametersSource=internal  P=0.8  I=0.1  D=0  N=100  InitialConditionSource=internal  InitialConditionForIntegrator=0  InitialConditionForFilter=0  ExternalReset=none  LimitOutput=off  UpperSaturationLimit=inf  LowerSaturationLimit=-inf  LinearizeAsGain=on  AntiWindupMode=none  Kb=1  TrackingMode=off  Kt=1  PParamMin=[]  PParamMax=[]  IParamMin=[]  IParamMax=[]  DParamMin=[]  DParamMax=[]  NParamMin=[]  NParamMax=[]  KbParamMin=[]  KbParamMax=[]  KtParamMin=[]  KtParamMax=[]  POutMin=[]  POutMax=[]  IOutMin=[]  IOutMax=[]  DOutMin=[]  DOutMax=[]  NOutMin=[]  NOutMax=[]  KbOutMin=[]  KbOutMax=[]  KtOutMin=[]  KtOutMax=[]  IntegratorOutMin=[]  IntegratorOutMax=[]  FilterOutMin=[]  FilterOutMax=[]  SumOutMin=[]  SumOutMax=[]  SumI1OutMin=[]  SumI1OutMax=[]  SumI2OutMin=[]  SumI2OutMax=[]  SumI3OutMin=[]  SumI3OutMax=[]  SumDOutMin=[]  SumDOutMax=[]  SaturationOutMin=[]  SaturationOutMax=[]  IntegratorContinuousStateAttributes=''  IntegratorStateMustResolveToSignalObject=off  IntegratorRTWStateStorageClass=Auto  FilterContinuousStateAttributes=''  FilterStateMustResolveToSignalObject=off  FilterRTWStateStorageClass=Auto  DifferentiatorICPrevScaledInput=0  DifferentiatorOutMin=[]  DifferentiatorOutMax=[]
  Reference Position and Direction in Global CS with variable Look Ahead : Subsystem
  Sum4 : Sum  Inputs=+--
  Sum5 : Sum  Inputs=|+-
  Switch : Switch  Criteria=u2 > Threshold
  Switch1 : Switch  Criteria=u2 > Threshold
  Switch2 : Switch  Criteria=u2 > Threshold
  To Workspace : ToWorkspace  VariableName=steer_latPID  SaveFormat=Timeseries  SampleTime=-1
  To Workspace1 : ToWorkspace  VariableName=steer_directPID  SaveFormat=Timeseries  SampleTime=-1
  To Workspace2 : ToWorkspace  VariableName=steer_steerPID  SaveFormat=Timeseries  SampleTime=-1
  Reference Steering Angle : Outport
  wires:
  Lateral Error/1(Lateral Error) -> PID Control Lateral Position/1  "Lateral Error"
  Sum5/1 -> PID Control Steering/1  "Delta Error"
  Estimated Position/1 -> " "/2
  " "/1 -> Lateral Error/2(Position Error (X,Y))  "Position Error"
  Reference Position and Direction in Global CS with variable Look Ahead/2(Position (X,Y)) -> " "/1
  Reference Position and Direction in Global CS with variable Look Ahead/1(Psi Sigma) -> Lateral Error/1(Psi Sigma), Sum4/1
  Sum4/1 -> PID Control Direction/1  "Delta Reference = Psi Sigma - Nu"
  Measured Steering Angle/1 -> Gain/1
  Estimated Heading/1 -> Sum4/3
  Measured Velocity/1 -> Reference Position and Direction in Global CS with variable Look Ahead/1(Velocity)
  Gain/1 -> Sum5/2
  Switch/1 -> Switch1/3, Sum4/2
  PID Control Lateral Position/1 -> To Workspace/1, Switch/1
  Constant/1 -> Switch/2
  Switch1/1 -> Switch2/3, Sum5/1
  PID Control Direction/1 -> To Workspace1/1, Switch1/1
  Constant1/1 -> Switch1/2
  PID Control Steering/1 -> To Workspace2/1, Switch2/1  "Delta Reference"
  Switch2/1 -> Reference Steering Angle/1
  Constant2/1 -> Switch2/2

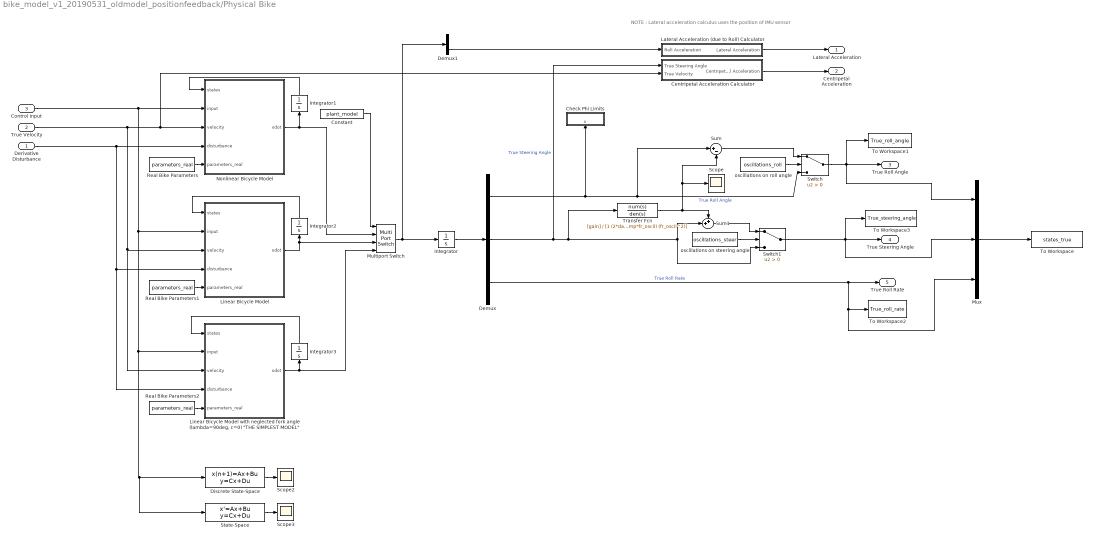
== system bike_model_v1_20190531_oldmodel_positionfeedback/Physical Bike ==
  note: NOTE : Lateral acceleration calculus uses the position of IMU sensor
  Derivative Disturbance : Inport
  True Velocity : Inport  Port=2
  Control Input : Inport  Port=3
  Centripetal Acceleration Calculator : Subsystem
  Check Phi Limits : Subsystem  TreatAsAtomicUnit=on  SystemSampleTime=Ts
  Constant : Constant  Value=plant_model
  Demux : Demux  Outputs=3
  Demux1 : Demux  Outputs=3
  Discrete State-Space : DiscreteStateSpace  A=sys_dis.A  B=sys_dis.B  C=eye(3,3)  D=zeros(3,1)  SampleTime=Ts_IMU
  Integrator{,1..3} (4 alike) : Integrator  InitialCondition=initial_states
  Lateral Acceleration (due to Roll) Calculator : Subsystem
  Linear Bicycle Model : MATLAB Function  TreatAsAtomicUnit=on
  "Linear Bicycle Model with neglected fork angle (lambda=90deg, c=0) \"THE SIMPLEST MODEL\"" : MATLAB Function  TreatAsAtomicUnit=on
  Multiport Switch : MultiPortSwitch
  Mux : Mux  Inputs=3
  Nonlinear Bicycle Model : MATLAB Function  TreatAsAtomicUnit=on
  Real Bike Parameters : Constant  Value=parameters_real
  Real Bike Parameters1 : Constant  Value=parameters_real
  Real Bike Parameters2 : Constant  Value=parameters_real
  Scope : Scope
  Scope2 : Scope
  Scope3 : Scope
  State-Space : StateSpace  A=sys_con.A  B=sys_con.B  C=eye(3,3)  D=zeros(3,1)  X0=0
  Sum : Sum  Inputs=|+-
  Sum1 : Sum  Inputs=++|
  Switch : Switch  Criteria=u2 > Threshold
  Switch1 : Switch  Criteria=u2 > Threshold
  To Workspace : ToWorkspace  VariableName=states_true  SaveFormat=Timeseries  SampleTime=Ts
  To Workspace1 : ToWorkspace  VariableName=True_roll_angle  SaveFormat=Structure  SampleTime=Ts
  To Workspace2 : ToWorkspace  VariableName=True_roll_rate  SaveFormat=Structure  SampleTime=Ts
  To Workspace3 : ToWorkspace  VariableName=True_steering_angle  SaveFormat=Structure  SampleTime=-1
  Transfer Fcn : TransferFcn  Numerator=[gain]  Denominator=[1 (2*damp*fr_oscil) (fr_oscil^2)]
  "oscillations on roll angle " : Constant  Value=oscillations_roll
  oscillations on steering angle : Constant  Value=oscillations_steer
  Lateral Acceleration : Outport
  Centripetal Acceleration : Outport  Port=2
  True Roll Angle : Outport  Port=3
  True Steering Angle : Outport  Port=4
  True Roll Rate : Outport  Port=5
  wires:
  Derivative Disturbance/1 -> "Linear Bicycle Model with neglected fork angle (lambda=90deg, c=0) \"THE SIMPLEST MODEL\""/4(disturbance), Linear Bicycle Model/4(disturbance), Nonlinear Bicycle Model/4(disturbance)
  Centripetal Acceleration Calculator/1(Centripetal Acceleration) -> Centripetal Acceleration/1
  Lateral Acceleration (due to Roll) Calculator/1(Lateral Acceleration) -> Lateral Acceleration/1
  True Velocity/1 -> Centripetal Acceleration Calculator/2(True Velocity), Nonlinear Bicycle Model/3(velocity), "Linear Bicycle Model with neglected fork angle (lambda=90deg, c=0) \"THE SIMPLEST MODEL\""/3(velocity), Linear Bicycle Model/3(velocity)
  Demux/3 -> To Workspace2/1, Mux/3, True Roll Rate/1  "True Roll Rate"
  Real Bike Parameters/1 -> Nonlinear Bicycle Model/5(parameters_real)
  Nonlinear Bicycle Model/1(xdot) -> Integrator1/1, Multiport Switch/2
  Linear Bicycle Model/1(xdot) -> Integrator2/1, Multiport Switch/3
  Real Bike Parameters1/1 -> Linear Bicycle Model/5(parameters_real)
  Multiport Switch/1 -> Demux1/1, Integrator/1
  Constant/1 -> Multiport Switch/1
  "Linear Bicycle Model with neglected fork angle (lambda=90deg, c=0) \"THE SIMPLEST MODEL\""/1(xdot) -> Integrator3/1, Multiport Switch/4
  Real Bike Parameters2/1 -> "Linear Bicycle Model with neglected fork angle (lambda=90deg, c=0) \"THE SIMPLEST MODEL\""/5(parameters_real)
  Demux1/3 -> Lateral Acceleration (due to Roll) Calculator/1(Roll Acceleration)
  Integrator/1 -> Demux/1
  Integrator3/1 -> "Linear Bicycle Model with neglected fork angle (lambda=90deg, c=0) \"THE SIMPLEST MODEL\""/1(states)
  Integrator2/1 -> Linear Bicycle Model/1(states)
  Integrator1/1 -> Nonlinear Bicycle Model/1(states)
  Discrete State-Space/1 -> Scope2/1
  State-Space/1 -> Scope3/1
  Control Input/1 -> State-Space/1, Discrete State-Space/1, "Linear Bicycle Model with neglected fork angle (lambda=90deg, c=0) \"THE SIMPLEST MODEL\""/2(input), Linear Bicycle Model/2(input), Nonlinear Bicycle Model/2(input)
  Mux/1 -> To Workspace/1
  Sum/1 -> Switch/1
  Demux/2 -> Switch1/3, Sum1/2, Transfer Fcn/1, Centripetal Acceleration Calculator/1(True Steering Angle)  "True Steering Angle"
  Demux/1 -> Sum/1, Switch/3, Check Phi Limits/1(x)  "True Roll Angle"
  "oscillations on roll angle "/1 -> Switch/2
  Transfer Fcn/1 -> Sum1/1, Scope/1, Sum/2
  Switch/1 -> True Roll Angle/1, To Workspace1/1, Mux/1
  Sum1/1 -> Switch1/1
  Switch1/1 -> To Workspace3/1, True Steering Angle/1, Mux/2
  oscillations on steering angle/1 -> Switch1/2

== system bike_model_v1_20190531_oldmodel_positionfeedback/Position sensor TEMPORARY ==
  True Position : Inport
  Constant : Constant  Value=noise
  Noise on position measurement system : RandomNumber  Variance=noise_pos_meas  SampleTime=Ts
  Sum : Sum  Inputs=++|
  Switch : Switch  Criteria=u2 > Threshold
  To Workspace3 : ToWorkspace  VariableName=pos_meas  SaveFormat=Timeseries  SampleTime=-1
  Zero-Order Hold : ZeroOrderHold  SampleTime=Ts
  "Measured Position (X,Y) " : Outport
  wires:
  True Position/1 -> Switch/3, Sum/2
  Sum/1 -> Switch/1
  Noise on position measurement system/1 -> Sum/1
  Switch/1 -> Zero-Order Hold/1
  Constant/1 -> Switch/2
  Zero-Order Hold/1 -> To Workspace3/1, "Measured Position (X,Y) "/1

== system bike_model_v1_20190531_oldmodel_positionfeedback/Steering Encoder ==
  Steering Angle (State) : Inport
  Constant : Constant  Value=noise
  Noise on steering encoder : RandomNumber  Variance=noise_encoder  Seed=6  SampleTime=Ts
  Sum : Sum  Inputs=++|
  Switch : Switch  Criteria=u2 > Threshold
  Zero-Order Hold : ZeroOrderHold  SampleTime=Ts
  Steering Angle : Outport
  wires:
  Constant/1 -> Switch/2
  Sum/1 -> Switch/1
  Steering Angle (State)/1 -> Sum/2, Switch/3
  Switch/1 -> Zero-Order Hold/1
  Zero-Order Hold/1 -> Steering Angle/1
  Noise on steering encoder/1 -> Sum/1

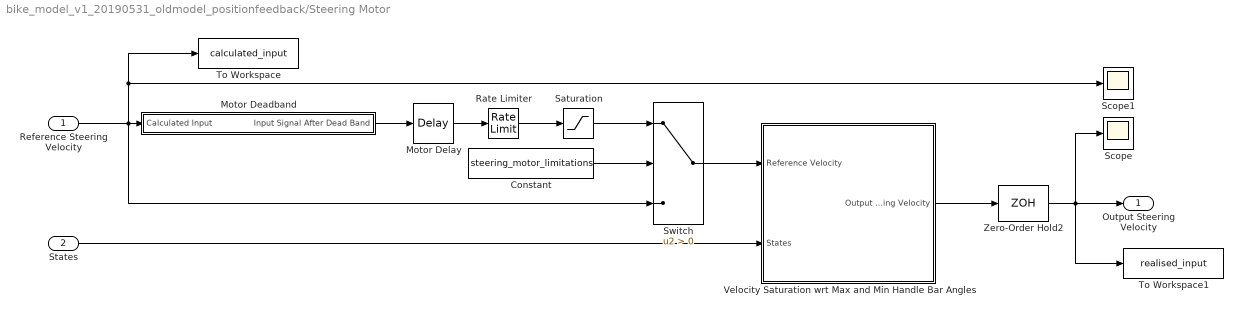
== system bike_model_v1_20190531_oldmodel_positionfeedback/Steering Motor ==
  Reference Steering Velocity : Inport
  States : Inport  Port=2
  Constant : Constant  Value=steering_motor_limitations
  Motor Delay : TransportDelay  DelayTime=delay
  Motor Deadband : Subsystem
  Rate Limiter : RateLimiter  RisingSlewLimit=max_steering_motor_acc  FallingSlewLimit=min_steering_motor_acc  SampleTimeMode=inherited
  Saturation : Saturate  UpperLimit=max_steering_motor_speed  LowerLimit=min_steering_motor_speed
  Scope : Scope
  Scope1 : Scope
  Switch : Switch  Criteria=u2 > Threshold
  To Workspace : ToWorkspace  VariableName=calculated_input  SaveFormat=Timeseries  SampleTime=Ts
  To Workspace1 : ToWorkspace  VariableName=realised_input  SaveFormat=Timeseries  SampleTime=Ts
  Velocity Saturation wrt Max and Min Handle Bar Angles : Subsystem
  Zero-Order Hold2 : ZeroOrderHold  SampleTime=Ts
  Output Steering Velocity : Outport
  wires:
  States/1 -> Velocity Saturation wrt Max and Min Handle Bar Angles/2(States)
  Motor Delay/1 -> Rate Limiter/1
  Constant/1 -> Switch/2
  Switch/1 -> Velocity Saturation wrt Max and Min Handle Bar Angles/1(Reference Velocity)
  Rate Limiter/1 -> Saturation/1
  Saturation/1 -> Switch/1
  Velocity Saturation wrt Max and Min Handle Bar Angles/1(Output Steering Velocity) -> Zero-Order Hold2/1
  Motor Deadband/1(Input Signal After Dead Band) -> Motor Delay/1
  Zero-Order Hold2/1 -> To Workspace1/1, Scope/1, Output Steering Velocity/1
  Reference Steering Velocity/1 -> Scope1/1, To Workspace/1, Motor Deadband/1(Calculated Input), Switch/3

== system bike_model_v1_20190531_oldmodel_positionfeedback/Velocity Reference ==
  note: If you will use this variable velocity
      | reference generator, you need to change
      | upper and lower limits of velocity specified
      | in initialization code!
  Add : Sum  Inputs=4
  Constant Velocity : Constant  Value=input_velocity
  Ramp : simulink/Sources/Ramp  slope=0.03  start=0  X0=0
  Reference Velocity Selector : ManualSwitch
  Sine Wave : Sin  Amplitude=0  SampleTime=0
  Step : Step  Time=20  Before=4  After=8  SampleTime=0
  Step1 : Step  Time=40  After=-1  SampleTime=0
  V_ref : Outport
  wires:
  Ramp/1 -> Add/4
  Constant Velocity/1 -> Reference Velocity Selector/1
  Step1/1 -> Add/3
  Step/1 -> Add/2
  Sine Wave/1 -> Add/1
  Add/1 -> Reference Velocity Selector/2
  Reference Velocity Selector/1 -> V_ref/1

== system bike_model_v1_20190531_oldmodel_positionfeedback/Balance Controller/LQR Controller ==
  note: Input = steering angular velocity
  Velocity : Inport
  State Error : Inport  Port=2
  1-D Lookup Table : Lookup_n-D  NumberOfTableDimensions=1  BreakpointsForDimension1=velocity_lqr  BreakpointsForDimension2=velocity_lqr  BreakpointsForDimension3=velocity_lqr  BreakpointsForDimension4=velocity_lqr  Table=K_full_dis(:,1)  InternalRulePriority=Speed  RndMeth=Simplest  InputSameDT=on
  1-D Lookup Table1 : Lookup_n-D  NumberOfTableDimensions=1  BreakpointsForDimension1=velocity_lqr  BreakpointsForDimension2=velocity_lqr  BreakpointsForDimension3=velocity_lqr  BreakpointsForDimension4=velocity_lqr  Table=K_full_dis(:,2)  InternalRulePriority=Speed  RndMeth=Simplest  InputSameDT=on
  1-D Lookup Table2 : Lookup_n-D  NumberOfTableDimensions=1  BreakpointsForDimension1=velocity_lqr  BreakpointsForDimension2=velocity_lqr  BreakpointsForDimension3=velocity_lqr  BreakpointsForDimension4=velocity_lqr  Table=K_full_dis(:,3)  InternalRulePriority=Speed  RndMeth=Simplest  InputSameDT=on
  Display1 : Display
  Mux : Mux  Inputs=3
  Product : Product  Multiplication=Matrix(*)
  Scope : Scope
  Transpose : Math  Operator=transpose  SaturateOnIntegerOverflow=on
  Zero-Order Hold : ZeroOrderHold  SampleTime=Ts
  Zero-Order Hold1 : ZeroOrderHold  SampleTime=Ts
  Calculated Input : Outport
  wires:
  1-D Lookup Table/1 -> Mux/1  "K1"
  1-D Lookup Table1/1 -> Mux/2  "K2"
  State Error/1 -> Zero-Order Hold1/1
  Product/1 -> Zero-Order Hold/1
  1-D Lookup Table2/1 -> Mux/3  "K3"
  Velocity/1 -> 1-D Lookup Table2/1, 1-D Lookup Table1/1, 1-D Lookup Table/1
  Mux/1 -> Product/2, Display1/1
  Transpose/1 -> Product/1
  Zero-Order Hold/1 -> Calculated Input/1
  Zero-Order Hold1/1 -> Scope/1, Transpose/1

== system bike_model_v1_20190531_oldmodel_positionfeedback/Balance Controller/Reference States ==
  Velocity : Inport
  Delta Ref : Inport  Port=2
  Bike Parameters : Constant  Value=parameters_real
  Constant : Constant  Value=path_tracking
  Mux5 : Mux  Inputs=3
  Reference Roll Angle Calculator : MATLAB Function  TreatAsAtomicUnit=on
  Switch : Switch  Criteria=u2 > Threshold
  Reference States : Outport
  wires:
  Bike Parameters/1 -> Reference Roll Angle Calculator/1(parameters_real)
  Switch/1 -> Mux5/2, Reference Roll Angle Calculator/3(delta_ref)
  Reference Roll Angle Calculator/1(phi_ref) -> Mux5/1
  Velocity/1 -> Reference Roll Angle Calculator/2(velocity)
  Mux5/1 -> Reference States/1
  Constant/1 -> Switch/2
  Delta Ref/1 -> Switch/1

== system bike_model_v1_20190531_oldmodel_positionfeedback/Complementary filter/Complementary Filter ==
  Roll Angle Estimation due to Accelerometer : Inport
  Roll Rate due to Gyroscope : Inport  Port=2
  Delay : Delay  DelayLength=1  InitialCondition=0
  Gain2 : Gain  Gain=complementary
  Gain3 : Gain  Gain=1-complementary
  Gain4 : Gain  Gain=Ts_IMU
  Sum3 : Sum  Inputs=|++
  Sum4 : Sum  Inputs=++|
  Roll Angle Estimation : Outport
  wires:
  Roll Angle Estimation due to Accelerometer/1 -> Gain3/1  "Roll_acc"
  Sum3/1 -> Gain2/1
  Roll Rate due to Gyroscope/1 -> Gain4/1
  Delay/1 -> Sum3/2
  Gain4/1 -> Sum3/1
  Gain2/1 -> Sum4/2
  Gain3/1 -> Sum4/1
  Sum4/1 -> Delay/1, Roll Angle Estimation/1
